simulink model "model_harmonic3"  (Simulink 7.0)
settings: Solver=ode45  StartTime=0.0  StopTime=10.0  MaxStep=0.1  RelTol=1e-3
settings Model: Creator=peter  LastModifiedBy=peter  ExtModeAutoUpdateStatusClock=off

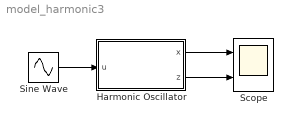
== system model_harmonic3 ==
  Harmonic Oscillator : Subsystem  mask(Harmonic oscillator){omega0=4, x0=0, v0=0, R=2e-4, seed=0, dt=0.05}
      mask prompts: omega0 "angular frequency"; x0 "initial displacement"; v0 "initial velocity"; R "variance of measurement"; seed "initial seed"; dt "sample time"
      mask help:
      | Linear oscillator
      | u:  control input
      | x: system output (x, v)
      | y: measurement output (x + W)
      mask Help:
      | Harmonic oscillator that is sampled with sample time dt
      | <ul>
      | <li>System output x: vector of position and velocity</li>
      | <li>Measurement output y: measurement of position x, including a normal
      |   random noise</li>
      | <li>Input u: control input, defining an external driving force</li>
      | </ul>
      mask Display:
      | plot(0:0.1:2*pi,sin(0:0.1:2*pi))
      | port_label('input', 1, 'u')
      | port_label('output', 1, 'x')
      | port_label('output', 2, 'z')
  Scope : Scope  NumInputPorts=2
      settings: TimeRange=10  YMin=-1~-0.4  YMax=1~0.4
  Sine Wave : Sin  Frequency=3  SampleTime=0
  wires:
  Sine Wave/1 -> Harmonic Oscillator/1(u)
  Harmonic Oscillator/2(z) -> Scope/2
  Harmonic Oscillator/1(x) -> Scope/1

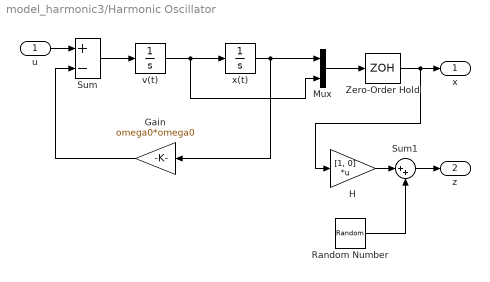
== system model_harmonic3/Harmonic Oscillator ==
  u : Inport
  Gain : Gain  Orientation=left  Gain=omega0*omega0  ParameterDataType=sfix(16)  ParameterScaling=2^0  OutDataType=sfix(16)  OutScaling=2^0
  H : Gain  Gain=[1, 0]  Multiplication=Matrix(K*u)  ParameterDataType=sfix(16)  ParameterScaling=2^0  OutDataType=sfix(16)  OutScaling=2^0
  Mux : Mux  Inputs=2
  Random Number : RandomNumber  Variance=R  Seed=seed  SampleTime=dt  VectorParams1D=off
  Sum : Sum  Inputs=+-  OutDataType=sfix(16)  OutScaling=2^0
  Sum1 : Sum  Inputs=|++  OutDataType=sfix(16)  OutScaling=2^0
  Zero-Order Hold : ZeroOrderHold  SampleTime=dt
  v(t) : Integrator  InitialCondition=v0
  x(t) : Integrator  InitialCondition=x0
  x : Outport
  z : Outport  Port=2
  wires:
  v(t)/1 -> x(t)/1, Mux/2
  x(t)/1 -> Gain/1, Mux/1
  Sum/1 -> v(t)/1
  Gain/1 -> Sum/2
  Mux/1 -> Zero-Order Hold/1
  Zero-Order Hold/1 -> H/1, x/1
  H/1 -> Sum1/1
  Random Number/1 -> Sum1/2
  u/1 -> Sum/1
  Sum1/1 -> z/1
